simulink model "centralized"  (R2017a)
settings: Solver=VariableStepAuto  StartTime=0.0  StopTime=6.01  RelTol=1e-3
values from neighbouring files (symbols this model uses):
  Kdd = diag(diagonald)    [calcula_ganhos.m]    (also in trajectoria_final.mat = [25.1327412287 0 0 0 0 0 0 25.1327412287 0 0 0 0 ... (36 ele; trajectoria_final_2speed.mat = [25.1327412287 0 0 0 0 0 0 25.1327412287 0 0 0 0 ... (36 ele; trajectoria_final_maxspeed.mat = [25.1327412287 0 0 0 0 0 0 25.1327412287 0 0 0 0 ... (36 ele)
  Kpp = diag (diagonalp)    [calcula_ganhos.m]    (also in trajectoria_final.mat = [157.913670417 0 0 0 0 0 0 157.913670417 0 0 0 0 ... (36 ele; trajectoria_final_2speed.mat = [157.913670417 0 0 0 0 0 0 157.913670417 0 0 0 0 ... (36 ele; trajectoria_final_maxspeed.mat = [157.913670417 0 0 0 0 0 0 157.913670417 0 0 0 0 ... (36 ele)
  q0 = [1.382 1.2 0.2 -0.5 0.4 0.34]'    [linear_trajectoryP.m]    (also in trajectoria_final.mat = [1.382 1.2 0.2 -0.5 0.4 0.34]; trajectoria_final_2speed.mat = [1.382 1.2 0.2 -0.5 0.4 0.34]; trajectoria_final_maxspeed.mat = [1.382 1.2 0.2 -0.5 0.4 0.34])
libraries: simulink x12, UR3_Lib x3, dspindex x2, sharedtransform x1, dspinverses x1
settings Model: Creator=dscat  LastModifiedBy=dscat

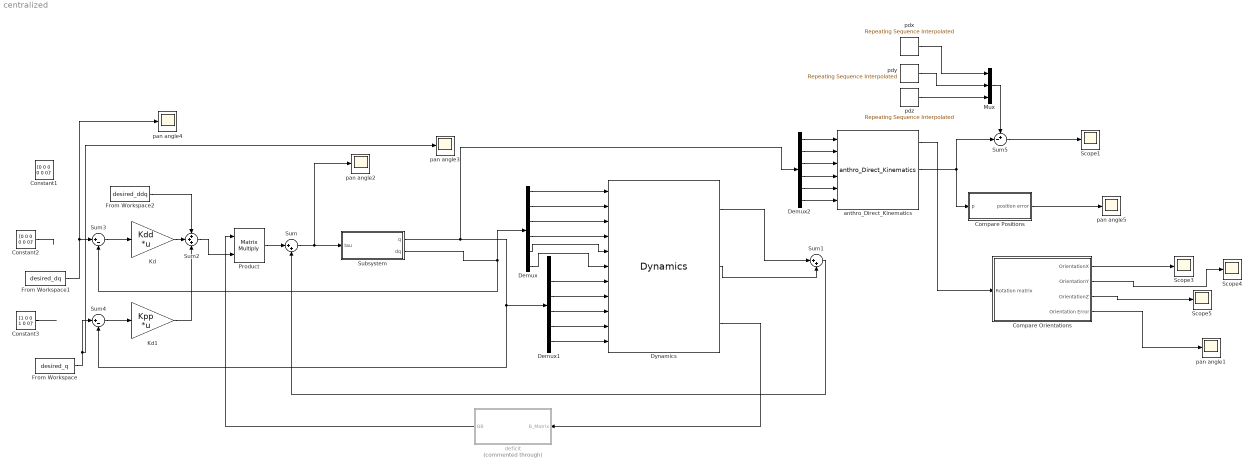
== system centralized ==
  Compare Orientations : Subsystem
  Compare Positions : Subsystem
  Constant1 : Constant  Value=[0 0 0 0 0 0]'
  Constant2 : Constant  Value=[0 0 0 0 0 0]'
  Constant3 : Constant  Value=[1 0 0 1 0 0]'
  Demux : Demux  Outputs=6
  Demux1 : Demux  Outputs=6
  Demux2 : Demux  Outputs=6
  Dynamics : UR3_Lib/Dynamics
  From Workspace : FromWorkspace  VariableName=desired_q  OutDataTypeStr=double  SampleTime=0
  From Workspace1 : FromWorkspace  VariableName=desired_dq  OutDataTypeStr=double  SampleTime=0
  From Workspace2 : FromWorkspace  VariableName=desired_ddq  OutDataTypeStr=double  SampleTime=0
  Kd : Gain  Gain=Kdd  Multiplication=Matrix(K*u)
  Kd1 : Gain  Gain=Kpp  Multiplication=Matrix(K*u)
  Mux : Mux  Inputs=3
  Product : Product  Multiplication=Matrix(*)
  Scope{1,3..5} (4 alike) : Scope
  Subsystem : Subsystem
  Sum : Sum  Inputs=|++
  Sum1 : Sum  Inputs=|++
  Sum2 : Sum  Inputs=+++
  Sum3 : Sum  Inputs=|+-
  Sum4 : Sum  Inputs=|+-
  Sum5 : Sum  Inputs=+-|
  anthro_Direct_Kinematics : UR3_Lib/anthro_Direct_Kinematics
  deficit : MATLAB Function  Commented=through  TreatAsAtomicUnit=on
  pan angle{1..5} (5 alike) : Scope
  pdx : simulink/Sources/Repeating Sequence Interpolated  OutValues=pdx  TimeValues=t  LookUpMeth=Interpolation-Use End Values  tsamp=0.01  OutMin=[]  OutMax=[]  OutDataTypeStr=double  OutputDataTypeScalingMode=double  OutDataType=fixdt(0,8)  OutScaling=2^-10
  pdy : simulink/Sources/Repeating Sequence Interpolated  OutValues=pdy  TimeValues=t  LookUpMeth=Interpolation-Use End Values  tsamp=0.01  OutMin=[]  OutMax=[]  OutDataTypeStr=double  OutputDataTypeScalingMode=double  OutDataType=fixdt(0,8)  OutScaling=2^-10
  pdz : simulink/Sources/Repeating Sequence Interpolated  OutValues=pdz  TimeValues=t  LookUpMeth=Interpolation-Use End Values  tsamp=0.01  OutMin=[]  OutMax=[]  OutDataTypeStr=double  OutputDataTypeScalingMode=double  OutDataType=fixdt(0,8)  OutScaling=2^-10
  wires:
  deficit/1(BB) -> Product/1
  Sum3/1 -> Kd/1
  Dynamics/3 -> deficit/1(B_Matrix)
  Subsystem/2(dq) -> Demux/1, Sum3/2
  Sum2/1 -> Product/2
  Product/1 -> Sum/1
  Dynamics/2 -> Sum1/2
  Dynamics/1 -> Sum1/1
  Kd/1 -> Sum2/2
  Sum4/1 -> Kd1/1
  Sum1/1 -> Sum/2
  Sum/1 -> pan angle2/1, Subsystem/1(tau)
  Constant2/1 -> ?
  Constant3/1 -> ?
  Kd1/1 -> Sum2/3
  Demux1/6 -> Dynamics/11
  Demux1/5 -> Dynamics/10
  Demux1/4 -> Dynamics/9
  Demux1/3 -> Dynamics/8
  Demux1/2 -> Dynamics/7
  Demux/6 -> Dynamics/6
  Demux/5 -> Dynamics/5
  Demux/4 -> Dynamics/4
  Demux/3 -> Dynamics/3
  Demux/2 -> Dynamics/2
  Demux/1 -> Dynamics/1
  From Workspace/1 -> pan angle3/1, Sum4/1
  From Workspace1/1 -> pan angle4/1, Sum3/1
  From Workspace2/1 -> Sum2/1
  Demux2/5 -> anthro_Direct_Kinematics/5
  Demux2/2 -> anthro_Direct_Kinematics/2
  anthro_Direct_Kinematics/2 -> Compare Positions/1("p "), Sum5/2
  Mux/1 -> Sum5/1
  Sum5/1 -> Scope1/1
  pdx/1 -> Mux/1
  Compare Positions/1(position error) -> pan angle5/1
  pdy/1 -> Mux/2
  Demux2/6 -> anthro_Direct_Kinematics/6
  Demux2/3 -> anthro_Direct_Kinematics/3
  Demux2/4 -> anthro_Direct_Kinematics/4
  Subsystem/1(q) -> Demux2/1, Demux1/1, Sum4/2
  Demux2/1 -> anthro_Direct_Kinematics/1
  pdz/1 -> Mux/3
  Compare Orientations/4(Orientation Error) -> pan angle1/1
  Compare Orientations/3(OrientationZ) -> Scope5/1
  Compare Orientations/2(OrientationY) -> Scope4/1
  Compare Orientations/1(OrientationX) -> Scope3/1
  anthro_Direct_Kinematics/1 -> Compare Orientations/1("Rotation matrix ")

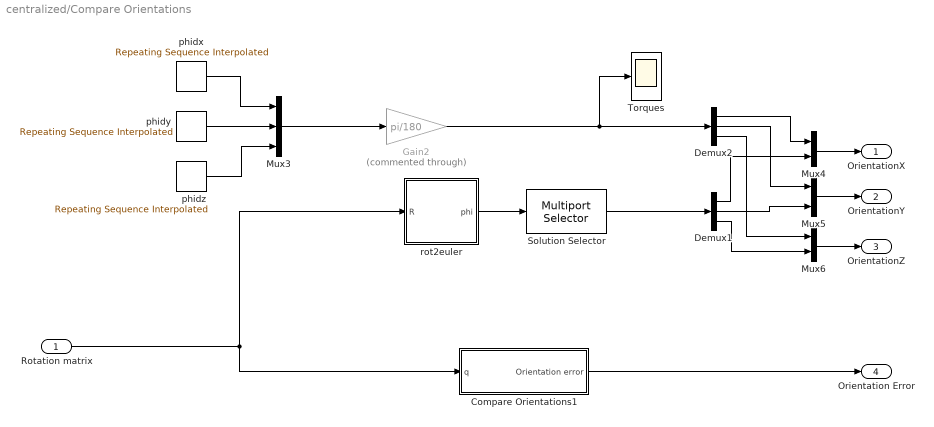
== system centralized/Compare Orientations ==
  "Rotation matrix " : Inport
  Compare Orientations1 : Subsystem
  Demux1 : Demux  Outputs=3
  Demux2 : Demux  Outputs=3
  Gain2 : Gain  Commented=through  Gain=pi/180
  Mux3 : Mux  Inputs=3
  Mux4 : Mux  Inputs=2
  Mux5 : Mux  Inputs=2
  Mux6 : Mux  Inputs=2
  Solution Selector : dspindex/Multiport Selector  rowsOrCols=Columns  idxCellArray=1  idxErrMode=Clip Index
  Torques : Scope
  phidx : simulink/Sources/Repeating Sequence Interpolated  OutValues=phidx  TimeValues=t  LookUpMeth=Interpolation-Use End Values  tsamp=0.01  OutMin=[]  OutMax=[]  OutDataTypeStr=double  OutputDataTypeScalingMode=double  OutDataType=fixdt(0,8)  OutScaling=2^-10
  phidy : simulink/Sources/Repeating Sequence Interpolated  OutValues=phidy  TimeValues=t  LookUpMeth=Interpolation-Use End Values  tsamp=0.01  OutMin=[]  OutMax=[]  OutDataTypeStr=double  OutputDataTypeScalingMode=double  OutDataType=fixdt(0,8)  OutScaling=2^-10
  phidz : simulink/Sources/Repeating Sequence Interpolated  OutValues=phidz  TimeValues=t  LookUpMeth=Interpolation-Use End Values  tsamp=0.01  OutMin=[]  OutMax=[]  OutDataTypeStr=double  OutputDataTypeScalingMode=double  OutDataType=fixdt(0,8)  OutScaling=2^-10
  rot2euler : MATLAB Function  TreatAsAtomicUnit=on
  OrientationX : Outport
  OrientationY : Outport  Port=2
  OrientationZ : Outport  Port=3
  Orientation Error : Outport  Port=4
  wires:
  Gain2/1 -> Demux2/1, Torques/1
  Compare Orientations1/1(Orientation error) -> Orientation Error/1
  phidx/1 -> Mux3/1
  Mux3/1 -> Gain2/1
  phidz/1 -> Mux3/3
  phidy/1 -> Mux3/2
  Mux6/1 -> OrientationZ/1
  Mux5/1 -> OrientationY/1
  Mux4/1 -> OrientationX/1
  Demux2/3 -> Mux6/1
  Demux2/2 -> Mux5/1
  Demux2/1 -> Mux4/1
  Demux1/1 -> Mux4/2
  Solution Selector/1 -> Demux1/1
  rot2euler/1(phi) -> Solution Selector/1
  Demux1/3 -> Mux6/2
  Demux1/2 -> Mux5/2
  "Rotation matrix "/1 -> Compare Orientations1/1("q "), rot2euler/1(R)

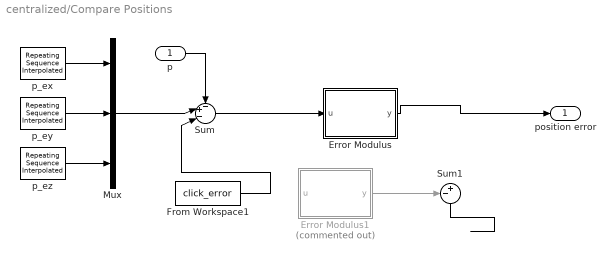
== system centralized/Compare Positions ==
  "p " : Inport
  Error Modulus : MATLAB Function  TreatAsAtomicUnit=on
  Error Modulus1 : MATLAB Function  Commented=on  TreatAsAtomicUnit=on
  From Workspace1 : FromWorkspace  VariableName=click_error  OutDataTypeStr=double  SampleTime=0
  Mux : Mux  Inputs=3
  Sum : Sum  Inputs=-+-|
  Sum1 : Sum  Inputs=-+|
  p_ex : simulink/Sources/Repeating Sequence Interpolated  OutValues=pdx  TimeValues=t  LookUpMeth=Interpolation-Use End Values  tsamp=0.01  OutMin=[]  OutMax=[]  OutDataTypeStr=double  OutputDataTypeScalingMode=double  OutDataType=fixdt(0,8)  OutScaling=2^-10
  p_ey : simulink/Sources/Repeating Sequence Interpolated  OutValues=pdy  TimeValues=t  LookUpMeth=Interpolation-Use End Values  tsamp=0.01  OutMin=[]  OutMax=[]  OutDataTypeStr=double  OutputDataTypeScalingMode=double  OutDataType=fixdt(0,8)  OutScaling=2^-10
  p_ez : simulink/Sources/Repeating Sequence Interpolated  OutValues=pdz  TimeValues=t  LookUpMeth=Interpolation-Use End Values  tsamp=0.01  OutMin=[]  OutMax=[]  OutDataTypeStr=double  OutputDataTypeScalingMode=double  OutDataType=fixdt(0,8)  OutScaling=2^-10
  position error : Outport
  wires:
  Sum/1 -> Error Modulus/1(u)
  "p "/1 -> Sum/1
  Error Modulus/1(y) -> position error/1
  Mux/1 -> Sum/2
  p_ez/1 -> Mux/3
  p_ey/1 -> Mux/2
  p_ex/1 -> Mux/1
  From Workspace1/1 -> Sum/3
  Error Modulus1/1(y) -> Sum1/1
  Sum1/1 -> ?

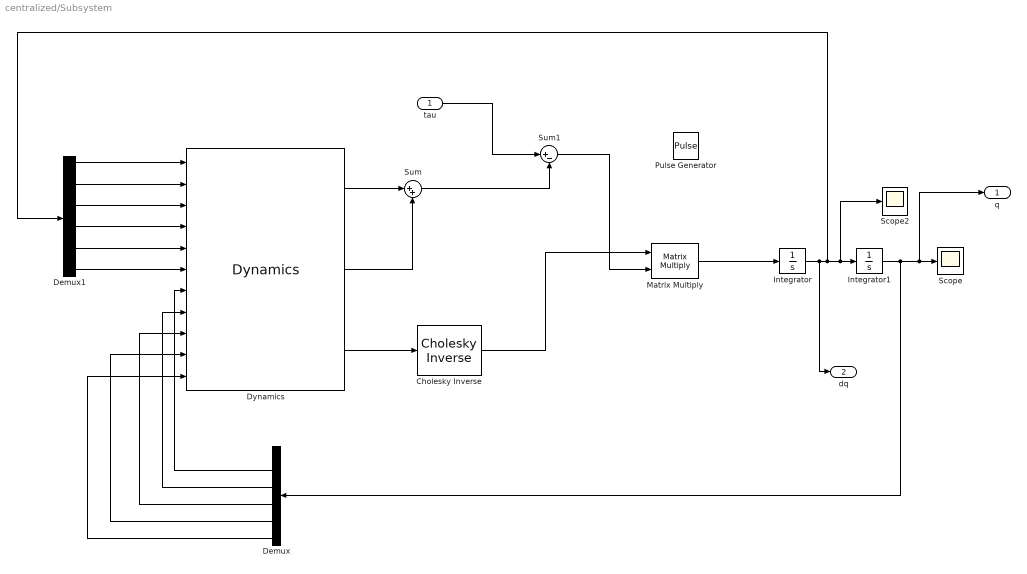
== system centralized/Subsystem ==
  tau : Inport
  Cholesky Inverse : dspinverses/Cholesky Inverse  errmode=Warning
      settings: SourceProductName=DSP System Toolbox  SourceProductBaseCode=DS
  Demux : Demux  Outputs=6
  Demux1 : Demux  Outputs=6
  Dynamics : UR3_Lib/Dynamics
  Integrator : Integrator  InitialCondition=[0 0 0 0 0 0]'
  Integrator1 : Integrator  InitialCondition=q0
  Matrix Multiply : Product  Multiplication=Matrix(*)
  Pulse Generator : DiscretePulseGenerator  PulseType=Time based  Amplitude=[1 0 0 0 0 0]  Period=3  PulseWidth=5
  Scope : Scope
  Scope2 : Scope
  Sum : Sum  Inputs=|++
  Sum1 : Sum  Inputs=|+-
  q : Outport
  dq : Outport  Port=2
  wires:
  tau/1 -> Sum1/1
  Demux/3 -> Dynamics/8
  Demux/5 -> Dynamics/10
  Demux1/3 -> Dynamics/3
  Demux1/4 -> Dynamics/4
  Demux1/2 -> Dynamics/2
  Demux1/5 -> Dynamics/5
  Demux/2 -> Dynamics/7
  Demux/4 -> Dynamics/9
  Demux1/6 -> Dynamics/6
  Matrix Multiply/1 -> Integrator/1
  Sum1/1 -> Matrix Multiply/2
  Dynamics/3 -> Cholesky Inverse/1
  Demux/6 -> Dynamics/11
  Dynamics/1 -> Sum/1
  Cholesky Inverse/1 -> Matrix Multiply/1
  Integrator/1 -> dq/1, Demux1/1, Scope2/1, Integrator1/1
  Sum/1 -> Sum1/2
  Dynamics/2 -> Sum/2
  Demux1/1 -> Dynamics/1
  Integrator1/1 -> Demux/1, q/1, Scope/1

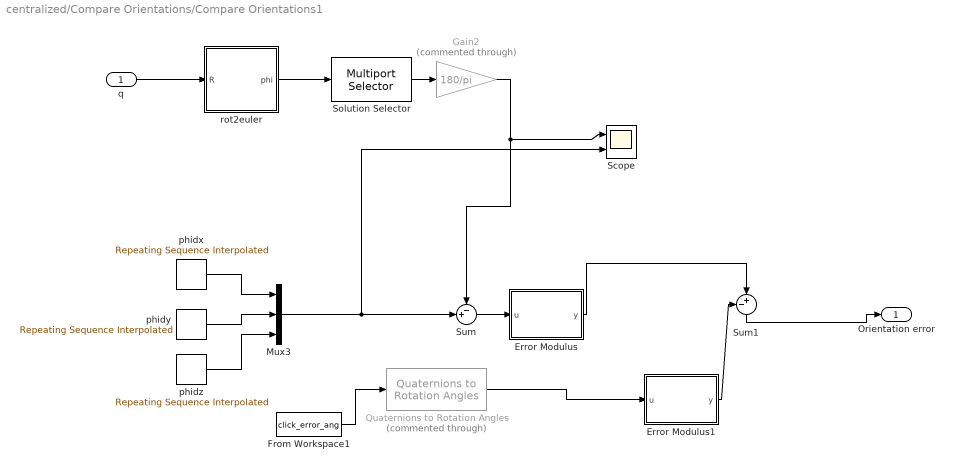
== system centralized/Compare Orientations/Compare Orientations1 ==
  "q " : Inport
  Error Modulus : MATLAB Function  TreatAsAtomicUnit=on
  Error Modulus1 : MATLAB Function  TreatAsAtomicUnit=on
  From Workspace1 : FromWorkspace  VariableName=click_error_ang  OutDataTypeStr=double  SampleTime=0
  Gain2 : Gain  Commented=through  Gain=180/pi
  Mux3 : Mux  Inputs=3
  Quaternions to Rotation Angles : sharedtransform/Quaternions to Rotation Angles  Commented=through  rotationOrder=ZYX
  Scope : Scope  NumInputPorts=2
  Solution Selector : dspindex/Multiport Selector  rowsOrCols=Columns  idxCellArray=1  idxErrMode=Clip Index
  Sum : Sum  Inputs=-+|
  Sum1 : Sum  Inputs=-+|
  phidx : simulink/Sources/Repeating Sequence Interpolated  OutValues=phidx  TimeValues=t  LookUpMeth=Interpolation-Use End Values  tsamp=0.01  OutMin=[]  OutMax=[]  OutDataTypeStr=double  OutputDataTypeScalingMode=double  OutDataType=fixdt(0,8)  OutScaling=2^-10
  phidy : simulink/Sources/Repeating Sequence Interpolated  OutValues=phidy  TimeValues=t  LookUpMeth=Interpolation-Use End Values  tsamp=0.01  OutMin=[]  OutMax=[]  OutDataTypeStr=double  OutputDataTypeScalingMode=double  OutDataType=fixdt(0,8)  OutScaling=2^-10
  phidz : simulink/Sources/Repeating Sequence Interpolated  OutValues=phidz  TimeValues=t  LookUpMeth=Interpolation-Use End Values  tsamp=0.01  OutMin=[]  OutMax=[]  OutDataTypeStr=double  OutputDataTypeScalingMode=double  OutDataType=fixdt(0,8)  OutScaling=2^-10
  rot2euler : MATLAB Function  TreatAsAtomicUnit=on
  Orientation error : Outport
  wires:
  Error Modulus/1(y) -> Sum1/2
  Gain2/1 -> Scope/1, Sum/1
  Sum/1 -> Error Modulus/1(u)
  Mux3/1 -> Sum/2, Scope/2
  Solution Selector/1 -> Gain2/1
  phidx/1 -> Mux3/1
  "q "/1 -> rot2euler/1(R)
  phidz/1 -> Mux3/3
  phidy/1 -> Mux3/2
  rot2euler/1(phi) -> Solution Selector/1
  From Workspace1/1 -> Quaternions to Rotation Angles/1
  Quaternions to Rotation Angles/1 -> Error Modulus1/1(u)
  Error Modulus1/1(y) -> Sum1/1
  Sum1/1 -> Orientation error/1

== matlab function centralized/Compare Orientations/Compare Orientations1/Error Modulus ==
  data: u input; y output
function y = Norm(u)
%#codegen

y = norm (u);

== matlab function centralized/Compare Orientations/Compare Orientations1/rot2euler ==
  data: R input; phi output
function phi   = Rot2Euler( R )
%This function converts the rotation matrix into Quarternion Representation
phi=zeros(3,2);

%phi_y6 € ]-pi/2,pi/2[
phi(1,1)=atan2(R(2,1),R(1,1));
phi(2,1)=atan2(-R(3,1),sqrt(R(3,2)^2+R(3,3)^2));
phi(3,1)=atan2(R(3,2),R(3,3));
%q6 € ]pi/2,3pi/2[
phi(1,2)=atan2(-R(2,1),-R(1,1));
phi(2,2)=atan2(-R(3,1),-sqrt(R(3,2)^2+R(3,3)^2));
phi(3,2)=atan2(-R(3,2),-R(3,3));

end

== matlab function centralized/Compare Orientations/Compare Orientations1/Error Modulus1 ==
  data: u input; y output
function y = Norm(u)
%#codegen

y = norm (u);

== matlab function centralized/Compare Positions/Error Modulus1 ==
  data: u input; y output
function y = Norm(u)
%#codegen

y = norm (u);

== matlab function centralized/Compare Orientations/rot2euler ==
  data: R input; phi output
function phi   = Rot2Euler( R )
%This function converts the rotation matrix into Quarternion Representation
phi=zeros(3,2);

%phi_y6 € ]-pi/2,pi/2[
phi(1,1)=atan2(R(2,1),R(1,1));
phi(2,1)=atan2(-R(3,1),sqrt(R(3,2)^2+R(3,3)^2));
phi(3,1)=atan2(R(3,2),R(3,3));
%q6 € ]pi/2,3pi/2[
phi(1,2)=atan2(-R(2,1),-R(1,1));
phi(2,2)=atan2(-R(3,1),-sqrt(R(3,2)^2+R(3,3)^2));
phi(3,2)=atan2(-R(3,2),-R(3,3));

end

== matlab function centralized/Compare Positions/Error Modulus ==
  data: u input; y output
function y = Norm(u)
%#codegen

y = norm (u);

== matlab function centralized/deficit ==
  data: B_Matrix input; BB output
function BB = Model_Error(B_Matrix)
%#codegen
BB=zeros(6);
deficit = 0.1;

BB = B_Matrix - deficit.*diag(diag(B_Matrix));
